simulink model "PIDMODEL"  (R2019b)
settings: Solver=ode4  StartTime=0.0  StopTime=inf  FixedStep=Ts  RelTol=1e-3  EnableMultiTasking=on
values from neighbouring files (symbols this model uses):
  Ts = 8    [matlab.mat]
libraries: arduino_io_lib x8, opclib x5, simulink x2, dspstat3 x1
settings Model: SILPILModeSetting=veronly  ExtModeTrigDuration=2  Creator=EK  LastModifiedBy=EK
settings SolverCC: AutoInsertRateTranBlk=on
settings DataIOCC: ReturnWorkspaceOutputs=off
settings OptimizationCC: EnhancedBackFolding=on  PassReuseOutputArgsAs=Individual arguments  ZeroExternalMemoryAtStartup=off  ZeroInternalMemoryAtStartup=off  MaxStackSize=64  OptimizeBlockOrder=speed  DifferentSizesBufferReuse=on  OptimizationCustomize=off  EfficientTunableParamExpr=on
settings DebuggingCC: ParameterTunabilityLossMsg=error  ArithmeticOperatorsInVariantConditions=warning
settings HardwareCC: ProdBitPerInt=16  ProdBitPerPointer=16  ProdBitPerSizeT=16  ProdBitPerPtrDiffT=16  ProdLargestAtomicFloat=None  ProdWordSize=8  ProdHWDeviceType=Atmel->AVR
settings SFSimCC: SimUseLocalCustomCode=off  MATLABDynamicMemAlloc=off  CustomCodeUndefinedFunction=UseInterfaceOnly
settings RTWCC: SystemTargetFile=ert.tlc  HardwareBoard=Arduino Uno  TLCOptions=-aInlineSetEventsForThisBaseRateFcn=TLC_FALSE -aSuppressMultiTaskScheduler=TLC_FALSE -aRateBasedStepFcn=1  TemplateMakefile=ert_default_tmf  GenerateReport=on  RTWUseLocalCustomCode=off  Toolchain=Arduino AVR  BuildConfiguration=Faster Runs  IncludeHyperlinkInReport=on  LaunchReport=on  GenerateTraceInfo=on  GenerateTraceReport=on  GenerateTraceReportSl=on  GenerateTraceReportSf=on  GenerateTraceReportEml=on
settings CodeAppCC: ForceParamTrailComments=on  IgnoreCustomStorageClasses=off  OperatorAnnotations=on  SimulinkDataObjDesc=on  SFDataObjDesc=on  InsertBlockDesc=on
settings ERTTargetCC: SupportContinuousTime=on  SupportVariableSizeSignals=on  ExtModeStaticAllocSize=250

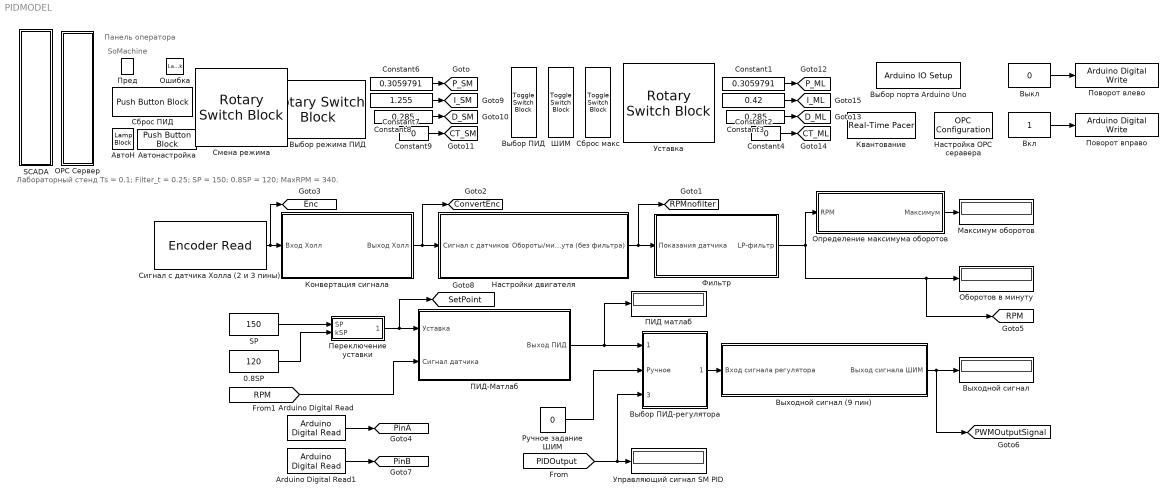
== system PIDMODEL ==
  note: Панель оператора
  note: Лабораторный стенд Ts = 0.1; Filter_t = 0.25; SP = 150; 0.8SP = 120; MaxRPM = 340.
  note: SoMachine
  0.8SP : Constant  Value=120
  Arduino Digital Read : arduino_io_lib/Arduino Digital Read  arduinoVar=Temporary arduino variable: Arduino1  arduinoPin=2  T=Ts
      settings: SourceProductName=Arduino IO Library
  Arduino Digital Read1 : arduino_io_lib/Arduino Digital Read  arduinoVar=Temporary arduino variable: Arduino1  arduinoPin=3  T=Ts
      settings: SourceProductName=Arduino IO Library
  Constant1 : Constant  Value=0.3059791
  Constant2 : Constant  Value=0.42
  Constant3 : Constant  Value=0.285
  Constant4 : Constant  Value=0
  Constant6 : Constant  Value=0.3059791
  Constant7 : Constant  Value=1.255
  Constant8 : Constant  Value=0.285
  Constant9 : Constant  Value=0
  OPC Сервер : Subsystem
  SCADA : Subsystem
  SP : Constant  Value=150
  АвтоН : LampBlock
  Автонастройка : PushButtonBlock  ButtonText=Автонастройка
  Вкл : Constant  SampleTime=-1
  Выбор ПИД : ToggleSwitchBlock
      settings: Values={{'SoMachine', 'Matlab'}, [0 1]}
  Выбор ПИД-регулятора : Subsystem
  Выбор порта Arduino Uno : arduino_io_lib/Arduino IO Setup  Priority=3  arduinoVar=Temporary arduino variable: Arduino1  workspaceVarName=a  comPort=COM5
      settings: SourceProductName=Arduino IO Library
  Выбор режима ПИД : RotarySwitchBlock
      settings: Values={{'Р', 'АН 1', 'АН 2', 'АН 3'}, [0 2 3 4]}
  Выкл : Constant  Value=0  SampleTime=-1
  Выходной сигнал : Display
  Выходной сигнал (9 пин) : Subsystem
  Квантование : arduino_io_lib/Real-Time Pacer  simTimePerRealTime=1
      settings: SourceProductName=Arduino IO Library
  Конвертация сигнала : Subsystem
  Максимум оборотов : Display
  Настройка OPC серавера : opclib/OPC Configuration  opcServers=localhost/CoDeSys.OPC.DA/10  errMissingItems=Error  errReadWrite=Warn  errShutdown=Error  errRTViolation=Warn  rtEnable=on  speedup=1  showLatency=off  beingUsed=on
      settings: SourceProductName=OPC Toolbox  SourceProductBaseCode=OT
  Настройки двигателя : Subsystem
  Оборотов в минуту : Display
  Определение максимума оборотов : Subsystem
  Ошибка : LampBlock
  ПИД матлаб : Display
  ПИД-Матлаб : Subsystem
  Переключение уставки : Subsystem
  Поворот влево : arduino_io_lib/Arduino Digital Write  arduinoVar=Temporary arduino variable: Arduino1  arduinoPin=4  T=0.1
      settings: SourceProductName=Arduino IO Library
  Поворот вправо : arduino_io_lib/Arduino Digital Write  arduinoVar=Temporary arduino variable: Arduino1  arduinoPin=5  T=0.1
      settings: SourceProductName=Arduino IO Library
  Пред : LampBlock
  Ручное задание ШИМ : Constant  Value=0
  Сброс ПИД : PushButtonBlock  ButtonText=Сброс ПИД
  Сброс макс : ToggleSwitchBlock
      settings: Values={{'Off', 'On'}, [0 1]}
  Сигнал с датчика Холла (2 и 3 пины) : arduino_io_lib/Encoder Read  arduinoVar=Temporary arduino variable: Arduino1  encNum=1  pinA=2  pinB=3  DbDl=0  T=Ts
      settings: SourceProductName=Arduino IO Library
  Смена режима : RotarySwitchBlock
      settings: Values={{'Ручной', 'Автомат'}, [0 1]}
  Управляющий сигнал SM PID : Display
  Уставка : RotarySwitchBlock
      settings: Values={{'0', '0.8SP', 'SP'}, [0 1 2]}
  Фильтр : Subsystem
  ШИМ : ToggleSwitchBlock
      settings: Values={{'0', '100%'}, [0 100]}
  tag scope: CT_ML=global, CT_SM=global, ConvertEnc=global, D_ML=global, D_SM=global, Enc=global, I_ML=global, I_SM=global, PWMOutputSignal=global, P_ML=global, P_SM=global, PinA=global, PinB=global, RPM=global, RPMnofilter=global, SetPoint=global
  wires:
  [PIDOutput] -> Выбор ПИД-регулятора/3(ПидSoMichine), Управляющий сигнал SM PID/1
  Сигнал с датчика Холла (2 и 3 пины)/1 -> [Enc], Конвертация сигнала/1(Вход Холл)
  ПИД-Матлаб/1(Выход ПИД) -> ПИД матлаб/1, Выбор ПИД-регулятора/1(ПидМатлаб)
  [RPM] -> ПИД-Матлаб/2(Сигнал датчика)
  Определение максимума оборотов/1(Максимум) -> Максимум оборотов/1
  Фильтр/1(LP-фильтр) -> [RPM], Оборотов в минуту/1, Определение максимума оборотов/1(RPM)
  Настройки двигателя/1(Обороты/минута (без фильтра)) -> [RPMnofilter], Фильтр/1(Показания датчика)
  SP/1 -> Переключение уставки/1(SP)
  0.8SP/1 -> Переключение уставки/2(kSP)
  Ручное задание ШИМ/1 -> Выбор ПИД-регулятора/2(Ручное)
  Выбор ПИД-регулятора/1(ВыходПИД) -> Выходной сигнал (9 пин)/1(Вход сигнала регулятора)
  Конвертация сигнала/1(Выход Холл) -> [ConvertEnc], Настройки двигателя/1(Сигнал с датчиков)
  Arduino Digital Read/1 -> [PinA]
  Arduino Digital Read1/1 -> [PinB]
  Переключение уставки/1(SPtoPID) -> [SetPoint], ПИД-Матлаб/1(Уставка)
  Constant6/1 -> [P_SM]
  Constant7/1 -> [I_SM]
  Constant8/1 -> [D_SM]
  Constant9/1 -> [CT_SM]
  Constant3/1 -> [D_ML]
  Constant1/1 -> [P_ML]
  Constant4/1 -> [CT_ML]
  Constant2/1 -> [I_ML]
  Вкл/1 -> Поворот вправо/1
  Выкл/1 -> Поворот влево/1
  Выходной сигнал (9 пин)/1(Выход сигнала ШИМ) -> [PWMOutputSignal], Выходной сигнал/1

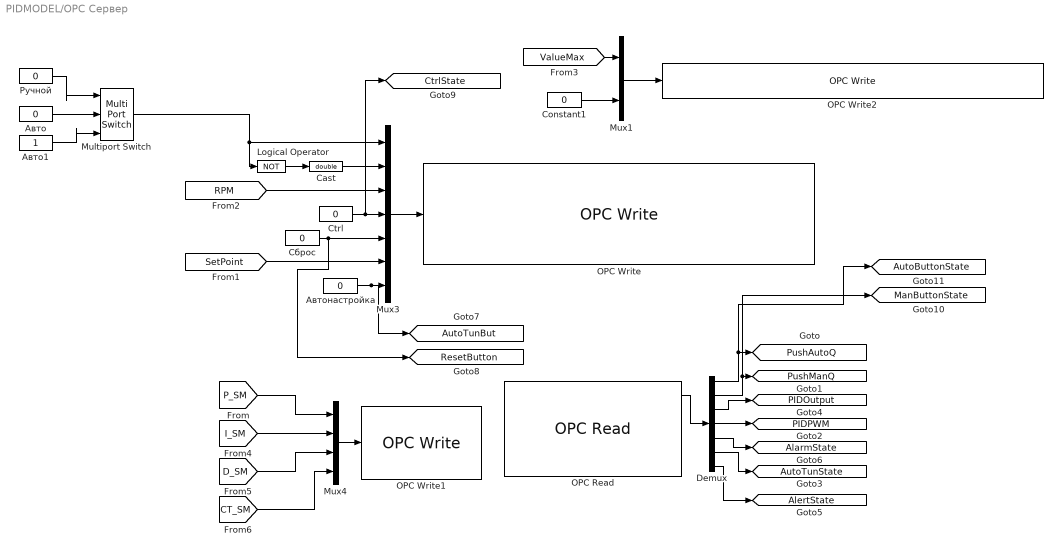
== system PIDMODEL/OPC Сервер ==
  Cast : DataTypeConversion  OutDataTypeStr=double
  Constant1 : Constant  Value=0
  Ctrl : Constant  Value=0
  Demux : Demux  Outputs=7
  Logical Operator : Logic  Operator=NOT  Inputs=1  AllPortsSameDT=off  OutDataTypeStr=boolean
  Multiport Switch : MultiPortSwitch  DataPortOrder=Zero-based contiguous  Inputs=2  zeroidx=on
  Mux1 : Mux  Inputs=2
  Mux3 : Mux  Inputs=7
  Mux4 : Mux
  OPC Read : opclib/OPC Read  serverHost=localhost  serverID=CoDeSys.OPC.DA  itemIDs=PLC_Id23.Application.GVL.Menu.PushAuto.Q1, PLC_Id23.Application.GVL.Menu.PushMan.Q1, PLC_Id23.Application.GVL.PID.OutputValue, PLC_Id23.Application.PERSISTENTVARS.ValveMem.PWM_Output, PLC_Id23.Application.GVL.PID.AlarmState, PLC_Id23.Application.GVL.PID.AutotuneState, PLC_Id23.Application.GVL.PID.AlertState  readMode=Synchronous (cache)  dataType=double  updateRate=0  showQual=on  showTS=on  tsMode=Seconds since start
      settings: SourceProductName=OPC Toolbox  SourceProductBaseCode=OT
  OPC Write : opclib/OPC Write  serverHost=localhost  serverID=CoDeSys.OPC.DA  itemIDs=PLC_Id23.Application.GVL.Menu.AutoButton, PLC_Id23.Application.GVL.Menu.ManButton, PLC_Id23.Application.PERSISTENTVARS.PIDMem.PV, PLC_Id23.Application.PERSISTENTVARS.PIDMem.CtrlMode, PLC_Id23.Application.GVL.Menu.ErrorResetButton, PLC_Id23.Application.PERSISTENTVARS.PIDMem.SP, PLC_Id23.Application.GVL.PID.AutoTunningButton  writeMode=Synchronous  updateRate=0
      settings: SourceProductName=OPC Toolbox  SourceProductBaseCode=OT
  OPC Write1 : opclib/OPC Write  serverHost=localhost  serverID=CoDeSys.OPC.DA  itemIDs=PLC_Id23.Application.PERSISTENTVARS.PIDMem.P, PLC_Id23.Application.PERSISTENTVARS.PIDMem.I, PLC_Id23.Application.PERSISTENTVARS.PIDMem.D, PLC_Id23.Application.PERSISTENTVARS.PIDMem.CT  writeMode=Synchronous  updateRate=0
      settings: SourceProductName=OPC Toolbox  SourceProductBaseCode=OT
  OPC Write2 : opclib/OPC Write  serverHost=localhost  serverID=CoDeSys.OPC.DA  itemIDs=PLC_Id23.Application.PERSISTENTVARS.PIDMem.TemperatureSetValueMax, PLC_Id23.Application.PERSISTENTVARS.PIDMem.TemperatureSetValueMin  writeMode=Synchronous  updateRate=0
      settings: SourceProductName=OPC Toolbox  SourceProductBaseCode=OT
  Авто : Constant  Value=0
  Авто1 : Constant
  Автонастройка : Constant  Value=0
  Ручной : Constant  Value=0
  Сброс : Constant  Value=0
  tag scope: AlarmState=global, AlertState=global, AutoButtonState=global, AutoTunBut=global, AutoTunState=global, CtrlState=global, ManButtonState=global, PIDOutput=global, PIDPWM=global, PushAutoQ=global, PushManQ=global, ResetButton=global
  wires:
  [D_SM] -> Mux4/3
  Demux/4 -> [PIDPWM]
  Mux4/1 -> OPC Write1/1
  OPC Read/1 -> Demux/1
  [CT_SM] -> Mux4/4
  [P_SM] -> Mux4/1
  Сброс/1 -> [ResetButton], Mux3/5
  [I_SM] -> Mux4/2
  Demux/2 -> [ManButtonState], [PushManQ]
  Mux3/1 -> OPC Write/1
  Demux/1 -> [AutoButtonState], [PushAutoQ]
  Demux/3 -> [PIDOutput]
  Автонастройка/1 -> [AutoTunBut], Mux3/7
  [SetPoint] -> Mux3/6
  [RPM] -> Mux3/3
  Demux/5 -> [AlarmState]
  Demux/6 -> [AutoTunState]
  Demux/7 -> [AlertState]
  Mux1/1 -> OPC Write2/1
  [ValueMax] -> Mux1/1
  Constant1/1 -> Mux1/2
  Ctrl/1 -> [CtrlState], Mux3/4
  Ручной/1 -> Multiport Switch/1
  Авто/1 -> Multiport Switch/2
  Авто1/1 -> Multiport Switch/3
  Multiport Switch/1 -> Logical Operator/1, Mux3/1
  Logical Operator/1 -> Cast/1
  Cast/1 -> Mux3/2

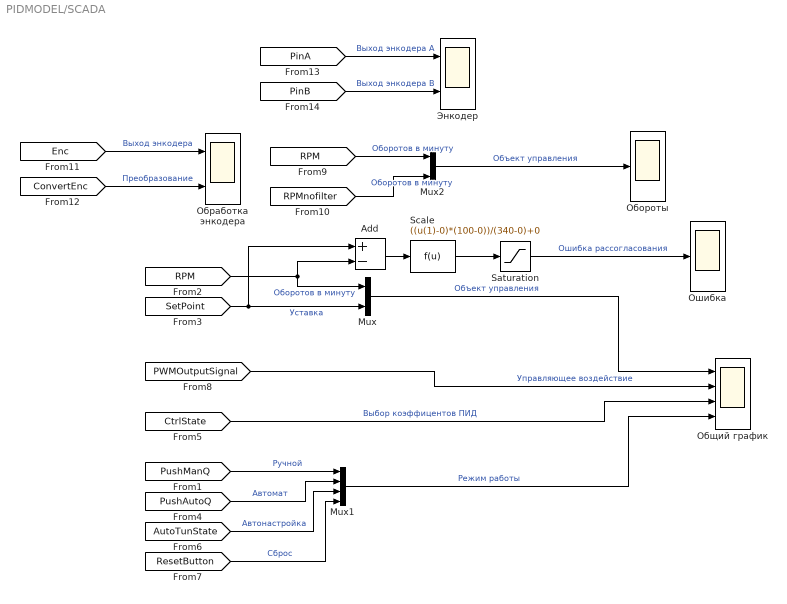
== system PIDMODEL/SCADA ==
  Add : Sum  Inputs=+-
  Mux : Mux  Inputs=2
  Mux1 : Mux
  Mux2 : Mux  Inputs=2
  Saturation : Saturate  UpperLimit=100  LowerLimit=0
  Scale : Fcn  Expr=((u(1)-0)*(100-0))/(340-0)+0
  Обороты : Scope
  Обработка энкодера : Scope  NumInputPorts=2
  Общий график : Scope  NumInputPorts=4
  Ошибка : Scope
  Энкодер : Scope  NumInputPorts=2
  wires:
  [RPM] -> Mux/1, Add/2  "Оборотов в минуту"
  [SetPoint] -> Mux/2, Add/1  "Уставка"
  Mux/1 -> Общий график/1  "Объект управления"
  [PushManQ] -> Mux1/1  "Ручной"
  [PushAutoQ] -> Mux1/2  "Автомат"
  [AutoTunState] -> Mux1/3  "Автонастройка"
  [ResetButton] -> Mux1/4  "Сброс"
  [CtrlState] -> Общий график/3  "Выбор коэффицентов ПИД"
  Mux1/1 -> Общий график/4  "Режим работы"
  Add/1 -> Scale/1
  Scale/1 -> Saturation/1
  Saturation/1 -> Ошибка/1  "Ошибка рассогласования"
  [RPM] -> Mux2/1  "Оборотов в минуту"
  [RPMnofilter] -> Mux2/2  "Оборотов в минуту"
  Mux2/1 -> Обороты/1  "Объект управления"
  [ConvertEnc] -> Обработка энкодера/2  "Преобразование"
  [Enc] -> Обработка энкодера/1  "Выход энкодера"
  [PinA] -> Энкодер/1  "Выход энкодера A"
  [PinB] -> Энкодер/2  "Выход энкодера B"
  [PWMOutputSignal] -> Общий график/2  "Управляющее воздействие"

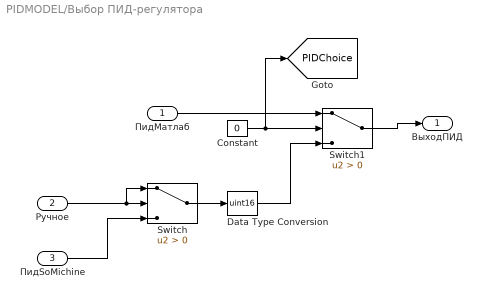
== system PIDMODEL/Выбор ПИД-регулятора ==
  ПидМатлаб : Inport
  Ручное : Inport  Port=2
  ПидSoMichine : Inport  Port=3
  Constant : Constant  Value=0
  Data Type Conversion : DataTypeConversion  OutDataTypeStr=uint16  SaturateOnIntegerOverflow=on
  Switch : Switch  Criteria=u2 > Threshold
  Switch1 : Switch  Criteria=u2 > Threshold
  ВыходПИД : Outport
  tag scope: PIDChoice=global
  wires:
  Ручное/1 -> Switch/1, Switch/2
  Switch/1 -> Data Type Conversion/1
  ПидSoMichine/1 -> Switch/3
  Data Type Conversion/1 -> Switch1/3
  Switch1/1 -> ВыходПИД/1
  ПидМатлаб/1 -> Switch1/1
  Constant/1 -> [PIDChoice], Switch1/2

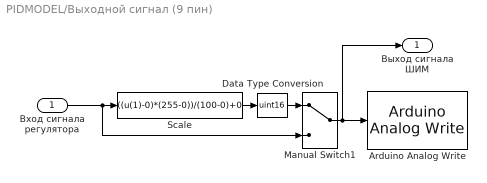
== system PIDMODEL/Выходной сигнал (9 пин) ==
  Вход сигнала регулятора : Inport
  Arduino Analog Write : arduino_io_lib/Arduino Analog Write  arduinoVar=Temporary arduino variable: Arduino1  arduinoPin=9  T=Ts
      settings: SourceProductName=Arduino IO Library
  Data Type Conversion : DataTypeConversion  OutDataTypeStr=uint16  SaturateOnIntegerOverflow=on
  Manual Switch1 : ManualSwitch
  Scale : Fcn  Expr=((u(1)-0)*(255-0))/(100-0)+0
  Выход сигнала ШИМ : Outport  VectorParamsAs1DForOutWhenUnconnected=off
  wires:
  Вход сигнала регулятора/1 -> Manual Switch1/2, Scale/1
  Scale/1 -> Data Type Conversion/1
  Manual Switch1/1 -> Выход сигнала ШИМ/1, Arduino Analog Write/1
  Data Type Conversion/1 -> Manual Switch1/1

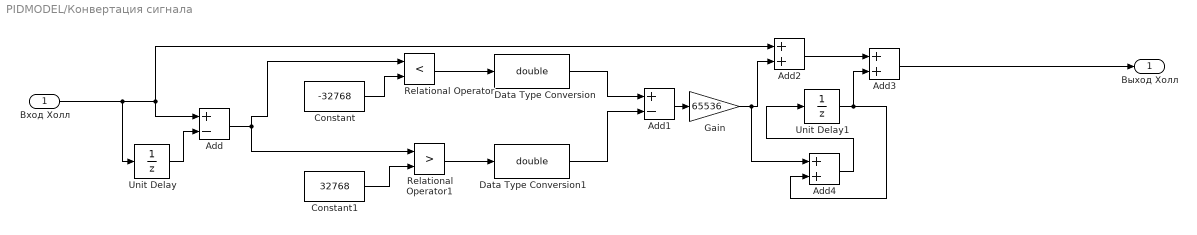
== system PIDMODEL/Конвертация сигнала ==
  Вход Холл : Inport
  Add : Sum  Inputs=+-
  Add1 : Sum  Inputs=+-
  Add2 : Sum
  Add3 : Sum
  Add4 : Sum
  Constant : Constant  Value=-32768
  Constant1 : Constant  Value=32768
  Data Type Conversion : DataTypeConversion  OutDataTypeStr=double
  Data Type Conversion1 : DataTypeConversion  OutDataTypeStr=double
  Gain : Gain  Gain=65536
  Relational Operator : RelationalOperator  Operator=<  OutDataTypeStr=boolean  RndMeth=Simplest
  Relational Operator1 : RelationalOperator  Operator=>  OutDataTypeStr=boolean  RndMeth=Simplest
  Unit Delay : UnitDelay  SampleTime=-1  HasFrameUpgradeWarning=on
  Unit Delay1 : UnitDelay  SampleTime=-1  HasFrameUpgradeWarning=on
  Выход Холл : Outport  OutDataTypeStr=double  VectorParamsAs1DForOutWhenUnconnected=off
  wires:
  Вход Холл/1 -> Add/1, Add2/1, Unit Delay/1
  Data Type Conversion/1 -> Add1/1
  Relational Operator1/1 -> Data Type Conversion1/1
  Unit Delay1/1 -> Add3/2, Add4/2
  Add1/1 -> Gain/1
  Gain/1 -> Add4/1, Add2/2
  Add2/1 -> Add3/1
  Add4/1 -> Unit Delay1/1
  Add/1 -> Relational Operator/1, Relational Operator1/1
  Relational Operator/1 -> Data Type Conversion/1
  Constant/1 -> Relational Operator/2
  Data Type Conversion1/1 -> Add1/2
  Constant1/1 -> Relational Operator1/2
  Unit Delay/1 -> Add/2
  Add3/1 -> Выход Холл/1

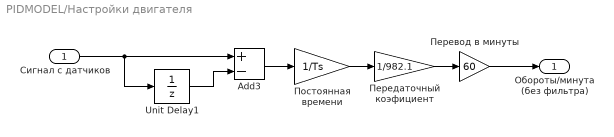
== system PIDMODEL/Настройки двигателя ==
  Сигнал с датчиков : Inport
  Add3 : Sum  Inputs=+-
  Unit Delay1 : UnitDelay  SampleTime=-1  HasFrameUpgradeWarning=on
  Перевод в минуты : Gain  Gain=60
  Передаточный коэфициент : Gain  Gain=1/982.1
  Постоянная времени : Gain  Gain=1/Ts
  Обороты/минута (без фильтра) : Outport  VectorParamsAs1DForOutWhenUnconnected=off
  wires:
  Сигнал с датчиков/1 -> Add3/1, Unit Delay1/1
  Add3/1 -> Постоянная времени/1
  Постоянная времени/1 -> Передаточный коэфициент/1
  Передаточный коэфициент/1 -> Перевод в минуты/1
  Unit Delay1/1 -> Add3/2
  Перевод в минуты/1 -> Обороты/минута (без фильтра)/1

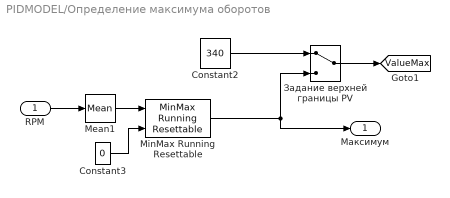
== system PIDMODEL/Определение максимума оборотов ==
  RPM : Inport
  Constant2 : Constant  Value=340
  Constant3 : Constant  Value=0
  Mean1 : dspstat3/Mean  run=off  InputProcessing=Columns as channels (frame based)  reset_popup=Rising edge  directionMode=Specified dimension  dimension=1  roiEnable=off  roiType=Rectangles  roiPortion=Entire ROI  roiOutput=Individual statistics for each ROI  roiFlag=off  roundingMode=Floor  overflowMode=off  outputDataTypeStr=Inherit: Same as accumulator  outputMin=[]  outputMax=[]  outputLastDataTypeStr=Inherit: Same as accumulator
  MinMax Running Resettable : simulink/Math Operations/MinMax Running Resettable  Function=max  vinit=0.0
  Задание верхней границы PV : ManualSwitch
  Максимум : Outport  VectorParamsAs1DForOutWhenUnconnected=off
  tag scope: ValueMax=global
  wires:
  Задание верхней границы PV/1 -> [ValueMax]
  MinMax Running Resettable/1 -> Максимум/1, Задание верхней границы PV/2
  Constant3/1 -> MinMax Running Resettable/2
  Constant2/1 -> Задание верхней границы PV/1
  Mean1/1 -> MinMax Running Resettable/1
  RPM/1 -> Mean1/1

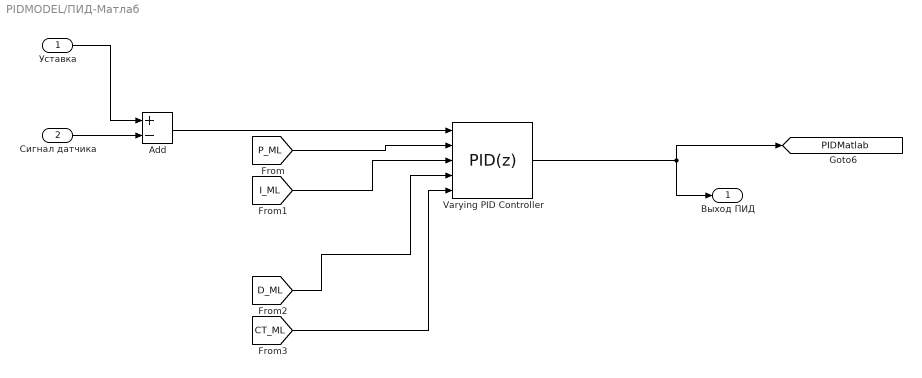
== system PIDMODEL/ПИД-Матлаб ==
  Уставка : Inport
  Сигнал датчика : Inport  Port=2
  Add : Sum  Inputs=+-
  Varying PID Controller : simulink/Continuous/PID Controller  Controller=PID  Form=Parallel  TimeDomain=Discrete-time  SampleTime=0.1  IntegratorMethod=Forward Euler  FilterMethod=Forward Euler  ControllerParametersSource=external  P=0.027559  I=0.42467  D=0.039006  UseFilter=on  N=3  TunerSelectOption=Frequency Response Based  InitialConditionSource=internal  InitialConditionForIntegrator=0  InitialConditionForFilter=0  DifferentiatorICPrevScaledInput=0  ExternalReset=none  TrackingMode=off  Kt=1  LimitOutput=on  UpperSaturationLimit=255  LowerSaturationLimit=0  LinearizeAsGain=off  AntiWindupMode=none  Kb=1  POutMin=[]  POutMax=[]  IOutMin=[]  IOutMax=[]  DOutMin=[]  DOutMax=[]  NOutMin=[]  NOutMax=[]  SumOutMin=[]  SumOutMax=[]  SaturationOutMin=[]  SaturationOutMax=[]  PParamMin=[]  PParamMax=[]  IParamMin=[]  IParamMax=[]  DParamMin=[]  DParamMax=[]  NParamMin=[]  NParamMax=[]  KbParamMin=[]  KbParamMax=[]  KtParamMin=[]  KtParamMax=[]  KbOutMin=[]  KbOutMax=[]  KtOutMin=[]  KtOutMax=[]  IntegratorOutMin=[]  IntegratorOutMax=[]  FilterOutMin=[]  FilterOutMax=[]  SumI1OutMin=[]  SumI1OutMax=[]  SumI2OutMin=[]  SumI2OutMax=[]  SumI3OutMin=[]  SumI3OutMax=[]  SumI4OutMin=[]  SumI4OutMax=[]  SumDOutMin=[]  SumDOutMax=[]  DifferentiatorOutMin=[]  DifferentiatorOutMax=[]  FilterDiffOutCoefMin=[]  FilterDiffOutCoefMax=[]  ReciprocalOutMin=[]  ReciprocalOutMax=[]  SumDenOutMin=[]  SumDenOutMax=[]  SumNumOutMin=[]  SumNumOutMax=[]  DivideOutMin=[]  DivideOutMax=[]  IntegratorContinuousStateAttributes=''  IntegratorStateMustResolveToSignalObject=off  IntegratorRTWStateStorageClass=Auto  FilterContinuousStateAttributes=''  FilterStateMustResolveToSignalObject=off  FilterRTWStateStorageClass=Auto  ParallelPVariant=ExternalParameters  IdealPVariant=Disabled  IVariant=ExternalParameters  DVariant=ExternalParameters  IntegratorVariant=Discrete  SatVariant=Enabled  AWVariant=Passthrough  PCopyVariant=Disabled  TRVariant=Disabled  FdbkBlocksVariant=Forward  IdealPFdbkVariant=Disabled  SatFdbkVariant=Disabled  DerivativeFilterVariant=ForwardEulerFilter  NVariant=ExternalParameters  NCopyVariant=Disabled  FilterICVariant=InternalICsFilter  IntegratorICVariant=InternalICs  ExternalResetVariant=Disabled  TRSumVariant=Passthrough  SumFdbkVariant=Disabled  SumVariant=Sum_PID
  Выход ПИД : Outport
  tag scope: PIDMatlab=global
  wires:
  Уставка/1 -> Add/1
  Сигнал датчика/1 -> Add/2
  [P_ML] -> Varying PID Controller/2
  [I_ML] -> Varying PID Controller/3
  [D_ML] -> Varying PID Controller/4
  [CT_ML] -> Varying PID Controller/5
  Varying PID Controller/1 -> Выход ПИД/1, [PIDMatlab]
  Add/1 -> Varying PID Controller/1

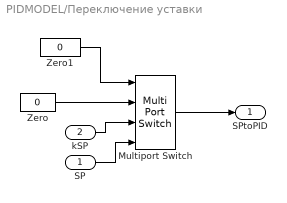
== system PIDMODEL/Переключение уставки ==
  SP : Inport
  kSP : Inport  Port=2
  Multiport Switch : MultiPortSwitch  DataPortOrder=Zero-based contiguous  zeroidx=on
  Zero : Constant  Value=0
  Zero1 : Constant  Value=0
  SPtoPID : Outport
  wires:
  Zero1/1 -> Multiport Switch/1
  kSP/1 -> Multiport Switch/3
  SP/1 -> Multiport Switch/4
  Zero/1 -> Multiport Switch/2
  Multiport Switch/1 -> SPtoPID/1

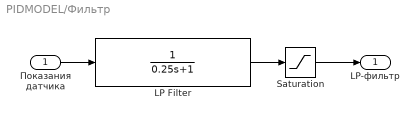
== system PIDMODEL/Фильтр ==
  Показания датчика : Inport
  LP Filter : TransferFcn  Denominator=[0.25 1]
  Saturation : Saturate  UpperLimit=340.0  LowerLimit=0.0
  LP-фильтр : Outport  VectorParamsAs1DForOutWhenUnconnected=off
  wires:
  Показания датчика/1 -> LP Filter/1
  LP Filter/1 -> Saturation/1
  Saturation/1 -> LP-фильтр/1
